simulink model "imu_model_with_submodules"  (R2015b)
settings: Solver=FixedStepAuto  StartTime=0.0  StopTime=10  FixedStep=1/mpu_sampling_frequency  RelTol=1e-3
values from neighbouring files (symbols this model uses):
  ex_acc_x = 0    [clipper.m]
  fs = mpu_sampling_frequency    [Madgwick_matlab.m]    (also in Mahony_matlab.m; clipper.m = 200)
  k = 0.05    [clipper.m]
  mpu_ax_noise_density = 300e-6    (= 0.0003)    [clipper.m]
  mpu_ax_sensitivity = 1/16384    (= 6.103515625e-05)    [clipper.m]
  mpu_ax_w = 460    [clipper.m]
  mpu_gyro_noise_density = 0.01    [clipper.m]
  mpu_gyro_sensitivity = 0.0610    (= 0.061)    [clipper.m]
  mpu_sampling_frequency = 200    [clipper.m]
  mpu_w = 250    [clipper.m]
undefined symbols (not defined in the file or in its folder): DiscIntNeverNeededParam, w_ax, wn, wn_ax, zeta, zeta_ax
libraries: simulink x9, aerolibtransform2 x2
settings Model: Creator=TOOsab  LastModifiedBy=TOOsab
settings DataIOCC: SaveOutput=off  SaveTime=off

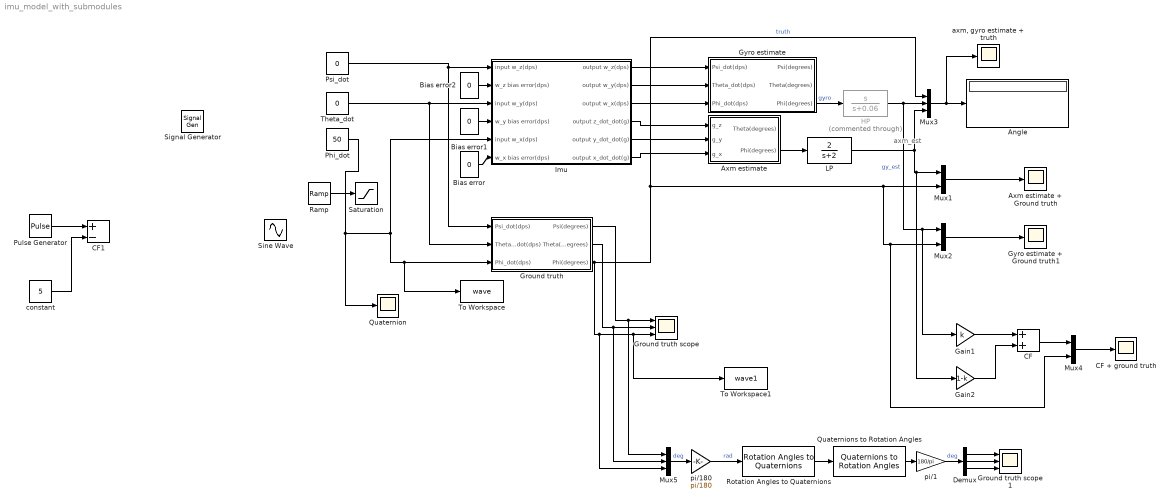
== system imu_model_with_submodules ==
  note: axm_est
  Angle : Display
  Axm estimate : Subsystem
  Axm estimate + Ground truth : Scope
  Bias error : Constant  Value=0
  Bias error1 : Constant  Value=0
  Bias error2 : Constant  Value=0
  CF : Sum
  CF + ground truth : Scope
  CF1 : Sum  Inputs=+-
  Demux : Demux  Outputs=3
  Gain1 : Gain  Gain=k
  Gain2 : Gain  Gain=1-k
  Ground truth : Subsystem
  "Ground truth scope " : Scope  NumInputPorts=3
  Ground truth scope 1 : Scope  NumInputPorts=3
  Gyro estimate : Subsystem
  Gyro estimate + Ground truth1 : Scope
  HP : TransferFcn  Commented=through  Numerator=[1 0]  Denominator=[1 0.06]
  Imu : Subsystem
  LP : TransferFcn  Numerator=[2]  Denominator=[1 2]
  Mux1 : Mux  Inputs=2
  Mux2 : Mux  Inputs=2
  Mux3 : Mux  Inputs=3
  Mux4 : Mux  Inputs=2
  Mux5 : Mux  Inputs=3
  Phi_dot : Constant  Value=50
  Psi_dot : Constant  Value=0
  Pulse Generator : DiscretePulseGenerator  PulseType=Time based  Amplitude=10  Period=10  PulseWidth=50
  Quaternion : Scope
  Quaternions to Rotation Angles : aerolibtransform2/Quaternions to Rotation Angles  rotationOrder=ZYX
  Ramp : simulink/Sources/Ramp  slope=1  start=1  X0=1
  Rotation Angles to Quaternions : aerolibtransform2/Rotation Angles to Quaternions  rotationOrder=ZYX
  Saturation : Saturate  UpperLimit=10
  Signal Generator : SignalGenerator  WaveForm=square  Frequency=0.1
  Sine Wave : Sin  Frequency=0.1  SampleTime=0
  Theta_dot : Constant  Value=0
  To Workspace : ToWorkspace  VariableName=wave  SampleTime=-1
  To Workspace1 : ToWorkspace  VariableName=wave1  SampleTime=-1
  "axm, gyro estimate + truth" : Scope
  constant : Constant  Value=5
  pi/1 : Gain  Gain=180/pi
  pi/180 : Gain  Gain=pi/180
  wires:
  Psi_dot/1 -> Ground truth/1(Psi_dot(dps)), Imu/1(input w_z(dps))
  Theta_dot/1 -> Ground truth/2(Theta_dot(dps)), Imu/3(input w_y(dps))
  Ramp/1 -> Saturation/1
  Imu/1(output w_z(dps)) -> Gyro estimate/1(Psi_dot(dps))
  Imu/2(output w_y(dps)) -> Gyro estimate/2(Theta_dot(dps))
  Imu/3(output w_x(dps)) -> Gyro estimate/3(Phi_dot(dps))
  Bias error/1 -> Imu/6(w_x bias error(dps))
  Ground truth/3(Phi(degrees)) -> Mux5/3, "Ground truth scope "/3, To Workspace1/1, Mux4/2, Mux2/2, Mux1/2, Mux3/1  "truth"
  Gyro estimate/3(Phi(degrees)) -> HP/1  "gyro"
  Mux3/1 -> Angle/1, "axm, gyro estimate + truth"/1
  Mux1/1 -> Axm estimate + Ground truth/1
  Bias error1/1 -> Imu/4(w_y bias error(dps))
  Bias error2/1 -> Imu/2(w_z bias error(dps))
  Imu/4(output z_dot_dot(g)) -> Axm estimate/1(g_z)
  Imu/5(output y_dot_dot(g)) -> Axm estimate/2(g_y)
  Imu/6(output x_dot_dot(g)) -> Axm estimate/3(g_x)
  Axm estimate/2(Phi(degrees)) -> LP/1
  LP/1 -> Gain2/1, Mux1/1, Mux3/3
  HP/1 -> Gain1/1, Mux2/1, Mux3/2  "gy_est"
  Mux2/1 -> Gyro estimate + Ground truth1/1
  Gain1/1 -> CF/1
  Gain2/1 -> CF/2
  CF/1 -> Mux4/1
  Mux4/1 -> CF + ground truth/1
  Ground truth/1(Psi(degrees)) -> "Ground truth scope "/1, Mux5/1
  Mux5/1 -> pi/180/1  "deg"
  Ground truth/2(Theta(degrees)) -> Mux5/2, "Ground truth scope "/2
  Rotation Angles to Quaternions/1 -> Quaternions to Rotation Angles/1
  Quaternions to Rotation Angles/1 -> pi/1/1
  Demux/1 -> Ground truth scope 1/1
  Demux/2 -> Ground truth scope 1/2
  Demux/3 -> Ground truth scope 1/3
  pi/180/1 -> Rotation Angles to Quaternions/1  "rad"
  pi/1/1 -> Demux/1  "deg"
  Phi_dot/1 -> Quaternion/1, Imu/5(input w_x(dps)), To Workspace/1, Ground truth/3(Phi_dot(dps))
  Pulse Generator/1 -> CF1/1
  constant/1 -> CF1/2

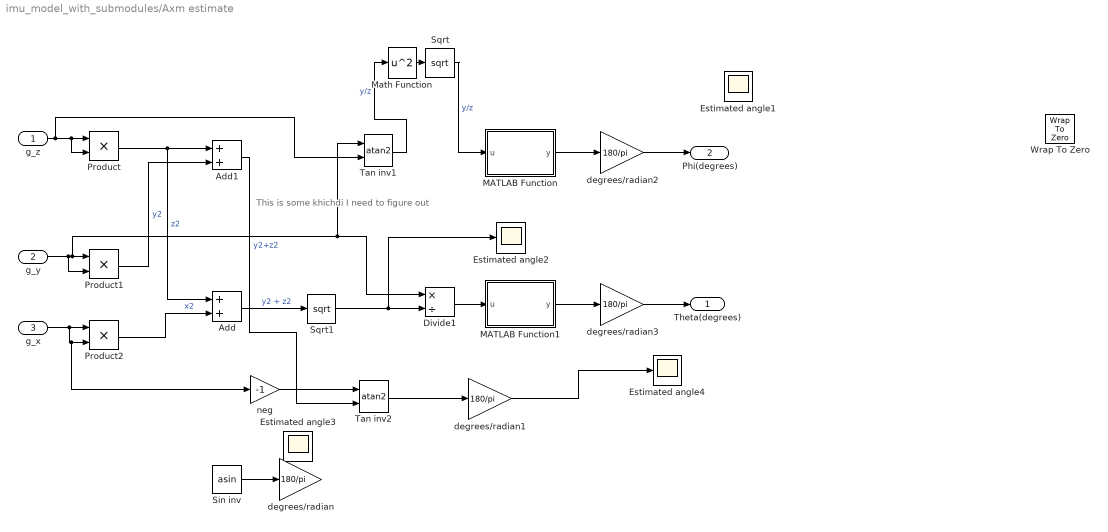
== system imu_model_with_submodules/Axm estimate ==
  note: This is some khichdi I need to figure out
  g_z : Inport
  g_y : Inport  Port=2
  g_x : Inport  Port=3
  Add : Sum
  Add1 : Sum
  Divide1 : Product  Inputs=*/
  Estimated angle{1..4} (4 alike) : Scope
  MATLAB Function : MATLAB Function  TreatAsAtomicUnit=on
  MATLAB Function1 : MATLAB Function  TreatAsAtomicUnit=on
  Math Function : Math  Operator=square  SaturateOnIntegerOverflow=on
  Product : Product
  Product1 : Product
  Product2 : Product
  Sin inv : Trigonometry  Operator=asin
  Sqrt : Sqrt  SaturateOnIntegerOverflow=on
  Sqrt1 : Sqrt  SaturateOnIntegerOverflow=on
  Tan inv1 : Trigonometry  Operator=atan2
  Tan inv2 : Trigonometry  Operator=atan2
  Wrap To Zero : simulink/Discontinuities/Wrap To Zero  Threshold=255
  degrees/radian{,1..3} (4 alike) : Gain  Gain=180/pi
  neg : Gain  Gain=-1
  Theta(degrees) : Outport
  Phi(degrees) : Outport  Port=2
  wires:
  Sin inv/1 -> degrees/radian/1
  g_z/1 -> Tan inv1/2, Product/2, Product/1
  g_y/1 -> Product1/2, Divide1/1, Tan inv1/1, Product1/1
  Product/1 -> Add/1, Add1/1  "z2"
  Product1/1 -> Add1/2  "y2"
  Product2/1 -> Add/2  "x2"
  Add/1 -> Sqrt1/1  "y2 + z2"
  Sqrt1/1 -> Estimated angle2/1, Divide1/2
  Divide1/1 -> MATLAB Function1/1(u)
  g_x/1 -> neg/1, Product2/2, Product2/1
  Add1/1 -> Tan inv2/2  "y2+z2"
  neg/1 -> Tan inv2/1
  Tan inv2/1 -> degrees/radian1/1
  degrees/radian1/1 -> Estimated angle4/1
  degrees/radian3/1 -> Theta(degrees)/1
  degrees/radian2/1 -> Phi(degrees)/1
  Sqrt/1 -> MATLAB Function/1(u)  "y/z"
  MATLAB Function/1(y) -> degrees/radian2/1
  MATLAB Function1/1(y) -> degrees/radian3/1
  Math Function/1 -> Sqrt/1
  Tan inv1/1 -> Math Function/1  "y/z"

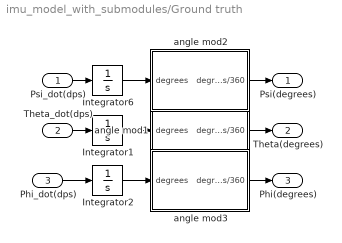
== system imu_model_with_submodules/Ground truth ==
  Psi_dot(dps) : Inport
  Theta_dot(dps) : Inport  Port=2
  Phi_dot(dps) : Inport  Port=3
  Integrator1 : Integrator
  Integrator2 : Integrator
  Integrator6 : Integrator
  angle mod1 : Subsystem
  angle mod2 : Subsystem
  angle mod3 : Subsystem
  Psi(degrees) : Outport
  Theta(degrees) : Outport  Port=2
  Phi(degrees) : Outport  Port=3
  wires:
  Phi_dot(dps)/1 -> Integrator2/1
  Integrator2/1 -> angle mod3/1(degrees)
  Theta_dot(dps)/1 -> Integrator1/1
  Psi_dot(dps)/1 -> Integrator6/1
  Integrator1/1 -> angle mod1/1(degrees)
  Integrator6/1 -> angle mod2/1(degrees)
  angle mod2/1(degrees/360) -> Psi(degrees)/1
  angle mod1/1(degrees/360) -> Theta(degrees)/1
  angle mod3/1(degrees/360) -> Phi(degrees)/1

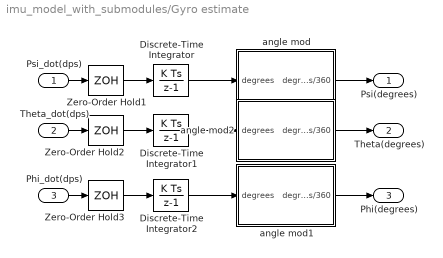
== system imu_model_with_submodules/Gyro estimate ==
  Psi_dot(dps) : Inport
  Theta_dot(dps) : Inport  Port=2
  Phi_dot(dps) : Inport  Port=3
  Discrete-Time Integrator : DiscreteIntegrator  InitialConditionSetting=State (most efficient)  SampleTime=1/mpu_sampling_frequency  ICPrevOutput=DiscIntNeverNeededParam  ICPrevScaledInput=DiscIntNeverNeededParam
  Discrete-Time Integrator1 : DiscreteIntegrator  InitialConditionSetting=State (most efficient)  SampleTime=1/mpu_sampling_frequency  ICPrevOutput=DiscIntNeverNeededParam  ICPrevScaledInput=DiscIntNeverNeededParam
  Discrete-Time Integrator2 : DiscreteIntegrator  InitialConditionSetting=State (most efficient)  SampleTime=1/mpu_sampling_frequency  ICPrevOutput=DiscIntNeverNeededParam  ICPrevScaledInput=DiscIntNeverNeededParam
  Zero-Order Hold1 : ZeroOrderHold  SampleTime=1/mpu_sampling_frequency
  Zero-Order Hold2 : ZeroOrderHold  SampleTime=1/mpu_sampling_frequency
  Zero-Order Hold3 : ZeroOrderHold  SampleTime=1/mpu_sampling_frequency
  angle mod : Subsystem
  angle mod1 : Subsystem
  angle mod2 : Subsystem
  Psi(degrees) : Outport
  Theta(degrees) : Outport  Port=2
  Phi(degrees) : Outport  Port=3
  wires:
  Zero-Order Hold1/1 -> Discrete-Time Integrator/1
  Zero-Order Hold3/1 -> Discrete-Time Integrator2/1
  Zero-Order Hold2/1 -> Discrete-Time Integrator1/1
  Discrete-Time Integrator2/1 -> angle mod1/1(degrees)
  Phi_dot(dps)/1 -> Zero-Order Hold3/1
  Discrete-Time Integrator/1 -> angle mod/1(degrees)
  Discrete-Time Integrator1/1 -> angle mod2/1(degrees)
  Psi_dot(dps)/1 -> Zero-Order Hold1/1
  Theta_dot(dps)/1 -> Zero-Order Hold2/1
  angle mod/1(degrees/360) -> Psi(degrees)/1
  angle mod2/1(degrees/360) -> Theta(degrees)/1
  angle mod1/1(degrees/360) -> Phi(degrees)/1

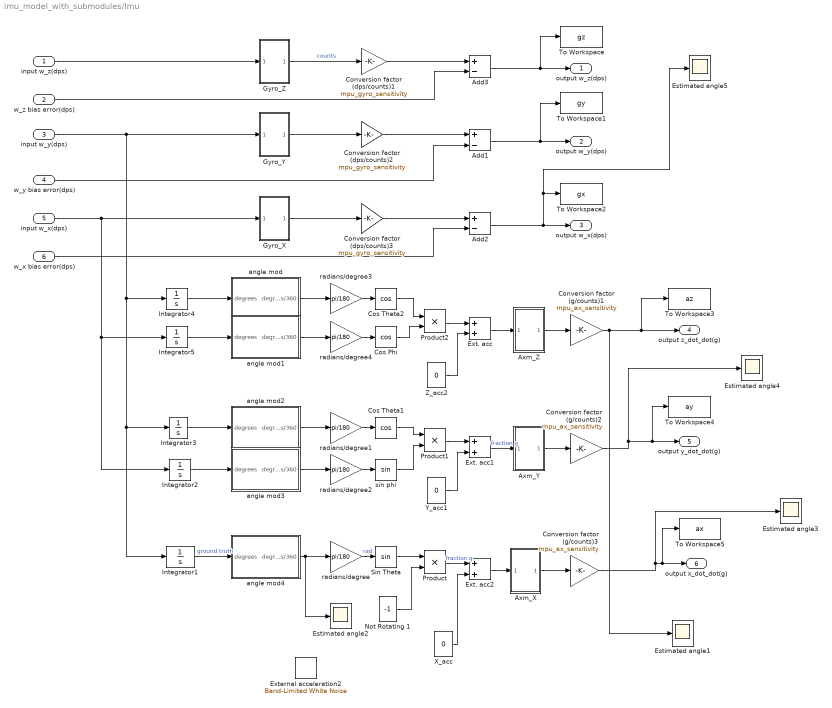
== system imu_model_with_submodules/Imu ==
  input w_z(dps) : Inport
  w_z bias error(dps) : Inport  Port=2
  input w_y(dps) : Inport  Port=3
  w_y bias error(dps) : Inport  Port=4
  input w_x(dps) : Inport  Port=5
  w_x bias error(dps) : Inport  Port=6
  Add1 : Sum  Inputs=+-
  Add2 : Sum  Inputs=+-
  Add3 : Sum  Inputs=+-
  Axm_X : Subsystem
  Axm_Y : Subsystem
  Axm_Z : Subsystem
  Conversion factor (dps/counts)1 : Gain  Gain=mpu_gyro_sensitivity
  Conversion factor (dps/counts)2 : Gain  Gain=mpu_gyro_sensitivity
  Conversion factor (dps/counts)3 : Gain  Gain=mpu_gyro_sensitivity
  Conversion factor (g/counts)1 : Gain  Gain=mpu_ax_sensitivity
  Conversion factor (g/counts)2 : Gain  Gain=mpu_ax_sensitivity
  Conversion factor (g/counts)3 : Gain  Gain=mpu_ax_sensitivity
  Cos Phi : Trigonometry  Operator=cos
  Cos Theta1 : Trigonometry  Operator=cos
  Cos Theta2 : Trigonometry  Operator=cos
  Estimated angle{1..5} (5 alike) : Scope
  Ext. acc : Sum
  Ext. acc1 : Sum
  Ext. acc2 : Sum
  External acceleration2 : simulink/Sources/Band-Limited White Noise  Cov=[ex_acc_x]  Ts=1/fs  seed=[23341]
  Gyro_X : Subsystem
  Gyro_Y : Subsystem
  Gyro_Z : Subsystem
  Integrator{1..5} (5 alike) : Integrator
  Not Rotating 1 : Constant  Value=-1
  Product : Product
  Product1 : Product
  Product2 : Product
  Sin Theta : Trigonometry
  To Workspace : ToWorkspace  VariableName=gz  SampleTime=-1
  To Workspace1 : ToWorkspace  VariableName=gy  SampleTime=-1
  To Workspace2 : ToWorkspace  VariableName=gx  SampleTime=-1
  To Workspace3 : ToWorkspace  VariableName=az  SampleTime=-1
  To Workspace4 : ToWorkspace  VariableName=ay  SampleTime=-1
  To Workspace5 : ToWorkspace  VariableName=ax  SampleTime=-1
  X_acc : Constant  Value=0
  Y_acc1 : Constant  Value=0
  Z_acc2 : Constant  Value=0
  angle mod : Subsystem
  angle mod1 : Subsystem
  angle mod2 : Subsystem
  angle mod3 : Subsystem
  angle mod4 : Subsystem
  radians/degree{,1..4} (5 alike) : Gain  Gain=pi/180
  sin phi : Trigonometry
  output w_z(dps) : Outport
  output w_y(dps) : Outport  Port=2
  output w_x(dps) : Outport  Port=3
  output z_dot_dot(g) : Outport  Port=4
  output y_dot_dot(g) : Outport  Port=5
  output x_dot_dot(g) : Outport  Port=6
  wires:
  input w_y(dps)/1 -> Integrator4/1, Integrator3/1, Integrator1/1, Gyro_Y/1(In1)
  Gyro_X/1(Out1) -> Conversion factor (dps/counts)3/1
  Gyro_Y/1(Out1) -> Conversion factor (dps/counts)2/1
  Gyro_Z/1(Out1) -> Conversion factor (dps/counts)1/1  "counts"
  input w_x(dps)/1 -> Integrator2/1, Integrator5/1, Gyro_X/1(In1)
  Conversion factor (dps/counts)2/1 -> Add1/1
  Add2/1 -> Estimated angle5/1, To Workspace2/1, output w_x(dps)/1
  Add3/1 -> To Workspace/1, output w_z(dps)/1
  Conversion factor (dps/counts)3/1 -> Add2/1
  Add1/1 -> To Workspace1/1, output w_y(dps)/1
  Conversion factor (dps/counts)1/1 -> Add3/1
  w_z bias error(dps)/1 -> Add3/2
  w_y bias error(dps)/1 -> Add1/2
  w_x bias error(dps)/1 -> Add2/2
  Integrator4/1 -> angle mod/1(degrees)
  radians/degree3/1 -> Cos Theta2/1
  Cos Theta2/1 -> Product2/1
  Integrator5/1 -> angle mod1/1(degrees)
  radians/degree4/1 -> Cos Phi/1
  Cos Phi/1 -> Product2/2
  Axm_Z/1(Out1) -> Conversion factor (g/counts)1/1
  Product2/1 -> Ext. acc/1
  Ext. acc1/1 -> Axm_Y/1(In1)  "fraction g"
  Axm_Y/1(Out1) -> Conversion factor (g/counts)2/1
  Integrator3/1 -> angle mod2/1(degrees)
  Integrator2/1 -> angle mod3/1(degrees)
  radians/degree1/1 -> Cos Theta1/1
  radians/degree2/1 -> sin phi/1
  Cos Theta1/1 -> Product1/1
  sin phi/1 -> Product1/2
  Sin Theta/1 -> Product/1
  Not Rotating 1/1 -> Product/2
  radians/degree/1 -> Sin Theta/1  "rad"
  Integrator1/1 -> angle mod4/1(degrees)  "ground truth"
  Axm_X/1(Out1) -> Conversion factor (g/counts)3/1
  Product/1 -> Ext. acc2/1  "fraction g"
  input w_z(dps)/1 -> Gyro_Z/1(In1)
  Conversion factor (g/counts)3/1 -> Estimated angle3/1, To Workspace5/1, output x_dot_dot(g)/1
  Conversion factor (g/counts)1/1 -> Estimated angle1/1, To Workspace3/1, output z_dot_dot(g)/1
  angle mod/1(degrees/360) -> radians/degree3/1
  angle mod1/1(degrees/360) -> radians/degree4/1
  angle mod2/1(degrees/360) -> radians/degree1/1
  angle mod3/1(degrees/360) -> radians/degree2/1
  angle mod4/1(degrees/360) -> Estimated angle2/1, radians/degree/1
  Conversion factor (g/counts)2/1 -> Estimated angle4/1, To Workspace4/1, output y_dot_dot(g)/1
  Ext. acc/1 -> Axm_Z/1(In1)
  Product1/1 -> Ext. acc1/1
  X_acc/1 -> Ext. acc2/2
  Ext. acc2/1 -> Axm_X/1(In1)
  Y_acc1/1 -> Ext. acc1/2
  Z_acc2/1 -> Ext. acc/2

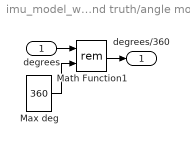
== system imu_model_with_submodules/Ground truth/angle mod1 ==
  degrees : Inport
  Math Function1 : Math  Operator=rem  RndMeth=Zero  SaturateOnIntegerOverflow=on
  Max deg : Constant  Value=360
  degrees/360 : Outport
  wires:
  degrees/1 -> Math Function1/1
  Max deg/1 -> Math Function1/2
  Math Function1/1 -> degrees/360/1

== system imu_model_with_submodules/Ground truth/angle mod2 ==
  degrees : Inport
  Math Function1 : Math  Operator=rem  RndMeth=Zero  SaturateOnIntegerOverflow=on
  Max deg : Constant  Value=360
  degrees/360 : Outport
  wires:
  degrees/1 -> Math Function1/1
  Max deg/1 -> Math Function1/2
  Math Function1/1 -> degrees/360/1

== system imu_model_with_submodules/Ground truth/angle mod3 ==
  degrees : Inport
  Math Function1 : Math  Operator=rem  RndMeth=Zero  SaturateOnIntegerOverflow=on
  Max deg : Constant  Value=360
  degrees/360 : Outport
  wires:
  degrees/1 -> Math Function1/1
  Max deg/1 -> Math Function1/2
  Math Function1/1 -> degrees/360/1

== system imu_model_with_submodules/Gyro estimate/angle mod ==
  degrees : Inport
  Math Function1 : Math  Operator=rem  RndMeth=Zero  SaturateOnIntegerOverflow=on
  Max deg : Constant  Value=360
  degrees/360 : Outport
  wires:
  degrees/1 -> Math Function1/1
  Max deg/1 -> Math Function1/2
  Math Function1/1 -> degrees/360/1

== system imu_model_with_submodules/Gyro estimate/angle mod1 ==
  degrees : Inport
  Math Function1 : Math  Operator=rem  RndMeth=Zero  SaturateOnIntegerOverflow=on
  Max deg : Constant  Value=360
  degrees/360 : Outport
  wires:
  degrees/1 -> Math Function1/1
  Max deg/1 -> Math Function1/2
  Math Function1/1 -> degrees/360/1

== system imu_model_with_submodules/Gyro estimate/angle mod2 ==
  degrees : Inport
  Math Function1 : Math  Operator=rem  RndMeth=Zero  SaturateOnIntegerOverflow=on
  Max deg : Constant  Value=360
  degrees/360 : Outport
  wires:
  degrees/1 -> Math Function1/1
  Max deg/1 -> Math Function1/2
  Math Function1/1 -> degrees/360/1

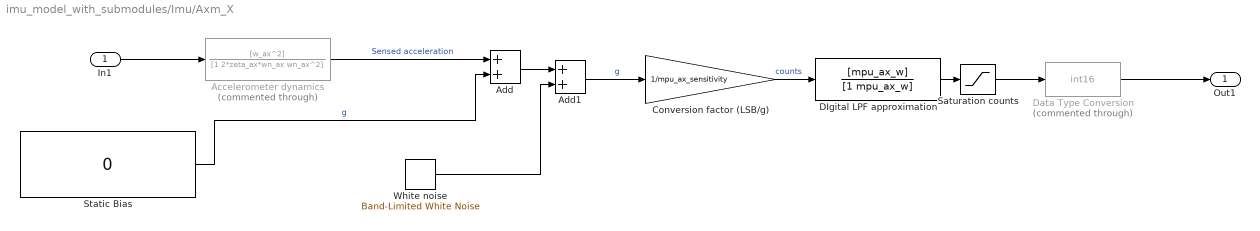
== system imu_model_with_submodules/Imu/Axm_X ==
  In1 : Inport
  Accelerometer dynamics : TransferFcn  Commented=through  Numerator=[w_ax^2]  Denominator=[1 2*zeta_ax*wn_ax wn_ax^2]
  Add : Sum
  Add1 : Sum
  Conversion factor (LSB/g) : Gain  Gain=1/mpu_ax_sensitivity
  DIgital LPF approximation : TransferFcn  Numerator=[mpu_ax_w]  Denominator=[1 mpu_ax_w]
  Data Type Conversion : DataTypeConversion  Commented=through  OutDataTypeStr=int16
  "Saturation counts " : Saturate  UpperLimit=2^15  LowerLimit=-2^15
  Static Bias : Constant  Value=0
  White noise : simulink/Sources/Band-Limited White Noise  Cov=[(mpu_ax_noise_density)^2]  Ts=1/mpu_sampling_frequency  seed=[23341]
  Out1 : Outport
  wires:
  In1/1 -> Accelerometer dynamics/1
  Data Type Conversion/1 -> Out1/1
  "Saturation counts "/1 -> Data Type Conversion/1
  DIgital LPF approximation/1 -> "Saturation counts "/1
  Add1/1 -> Conversion factor (LSB/g)/1  "g"
  Add/1 -> Add1/1
  White noise/1 -> Add1/2
  Accelerometer dynamics/1 -> Add/1  "Sensed acceleration"
  Static Bias/1 -> Add/2  "g"
  Conversion factor (LSB/g)/1 -> DIgital LPF approximation/1  "counts"

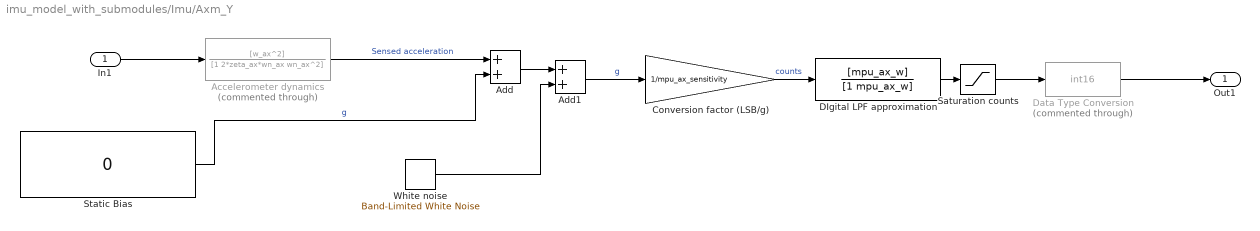
== system imu_model_with_submodules/Imu/Axm_Y ==
  In1 : Inport
  Accelerometer dynamics : TransferFcn  Commented=through  Numerator=[w_ax^2]  Denominator=[1 2*zeta_ax*wn_ax wn_ax^2]
  Add : Sum
  Add1 : Sum
  Conversion factor (LSB/g) : Gain  Gain=1/mpu_ax_sensitivity
  DIgital LPF approximation : TransferFcn  Numerator=[mpu_ax_w]  Denominator=[1 mpu_ax_w]
  Data Type Conversion : DataTypeConversion  Commented=through  OutDataTypeStr=int16
  "Saturation counts " : Saturate  UpperLimit=2^15  LowerLimit=-2^15
  Static Bias : Constant  Value=0
  White noise : simulink/Sources/Band-Limited White Noise  Cov=[(mpu_ax_noise_density)^2]  Ts=1/mpu_sampling_frequency  seed=[23341]
  Out1 : Outport
  wires:
  In1/1 -> Accelerometer dynamics/1
  Data Type Conversion/1 -> Out1/1
  "Saturation counts "/1 -> Data Type Conversion/1
  DIgital LPF approximation/1 -> "Saturation counts "/1
  Add1/1 -> Conversion factor (LSB/g)/1  "g"
  Add/1 -> Add1/1
  White noise/1 -> Add1/2
  Accelerometer dynamics/1 -> Add/1  "Sensed acceleration"
  Static Bias/1 -> Add/2  "g"
  Conversion factor (LSB/g)/1 -> DIgital LPF approximation/1  "counts"

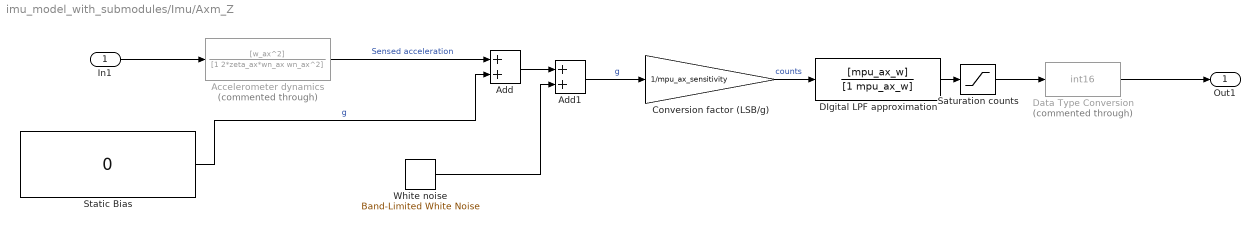
== system imu_model_with_submodules/Imu/Axm_Z ==
  In1 : Inport
  Accelerometer dynamics : TransferFcn  Commented=through  Numerator=[w_ax^2]  Denominator=[1 2*zeta_ax*wn_ax wn_ax^2]
  Add : Sum
  Add1 : Sum
  Conversion factor (LSB/g) : Gain  Gain=1/mpu_ax_sensitivity
  DIgital LPF approximation : TransferFcn  Numerator=[mpu_ax_w]  Denominator=[1 mpu_ax_w]
  Data Type Conversion : DataTypeConversion  Commented=through  OutDataTypeStr=int16
  "Saturation counts " : Saturate  UpperLimit=2^15  LowerLimit=-2^15
  Static Bias : Constant  Value=0
  White noise : simulink/Sources/Band-Limited White Noise  Cov=[(mpu_ax_noise_density)^2]  Ts=1/mpu_sampling_frequency  seed=[23341]
  Out1 : Outport
  wires:
  In1/1 -> Accelerometer dynamics/1
  Data Type Conversion/1 -> Out1/1
  "Saturation counts "/1 -> Data Type Conversion/1
  DIgital LPF approximation/1 -> "Saturation counts "/1
  Add1/1 -> Conversion factor (LSB/g)/1  "g"
  Add/1 -> Add1/1
  White noise/1 -> Add1/2
  Accelerometer dynamics/1 -> Add/1  "Sensed acceleration"
  Static Bias/1 -> Add/2  "g"
  Conversion factor (LSB/g)/1 -> DIgital LPF approximation/1  "counts"

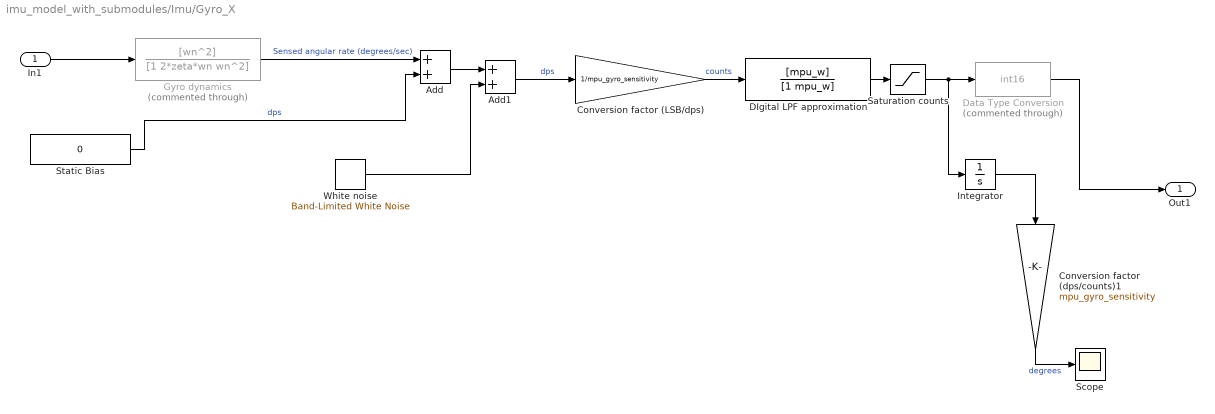
== system imu_model_with_submodules/Imu/Gyro_X ==
  In1 : Inport
  Add : Sum
  Add1 : Sum
  Conversion factor (LSB/dps) : Gain  Gain=1/mpu_gyro_sensitivity
  Conversion factor (dps/counts)1 : Gain  Gain=mpu_gyro_sensitivity
  DIgital LPF approximation : TransferFcn  Numerator=[mpu_w]  Denominator=[1 mpu_w]
  Data Type Conversion : DataTypeConversion  Commented=through  OutDataTypeStr=int16
  Gyro dynamics : TransferFcn  Commented=through  Numerator=[wn^2]  Denominator=[1 2*zeta*wn wn^2]
  Integrator : Integrator
  "Saturation counts " : Saturate  UpperLimit=2^15  LowerLimit=-2^15
  Scope : Scope
  Static Bias : Constant  Value=0
  White noise : simulink/Sources/Band-Limited White Noise  Cov=[(mpu_gyro_noise_density)^2]  Ts=1/mpu_sampling_frequency  seed=[23341]
  Out1 : Outport
  wires:
  Gyro dynamics/1 -> Add/1  "Sensed angular rate (degrees/sec)"
  White noise/1 -> Add1/2
  Static Bias/1 -> Add/2  "dps"
  Conversion factor (LSB/dps)/1 -> DIgital LPF approximation/1  "counts"
  Add/1 -> Add1/1
  Conversion factor (dps/counts)1/1 -> Scope/1  "degrees"
  Integrator/1 -> Conversion factor (dps/counts)1/1
  Data Type Conversion/1 -> Out1/1
  In1/1 -> Gyro dynamics/1
  "Saturation counts "/1 -> Integrator/1, Data Type Conversion/1
  DIgital LPF approximation/1 -> "Saturation counts "/1
  Add1/1 -> Conversion factor (LSB/dps)/1  "dps"

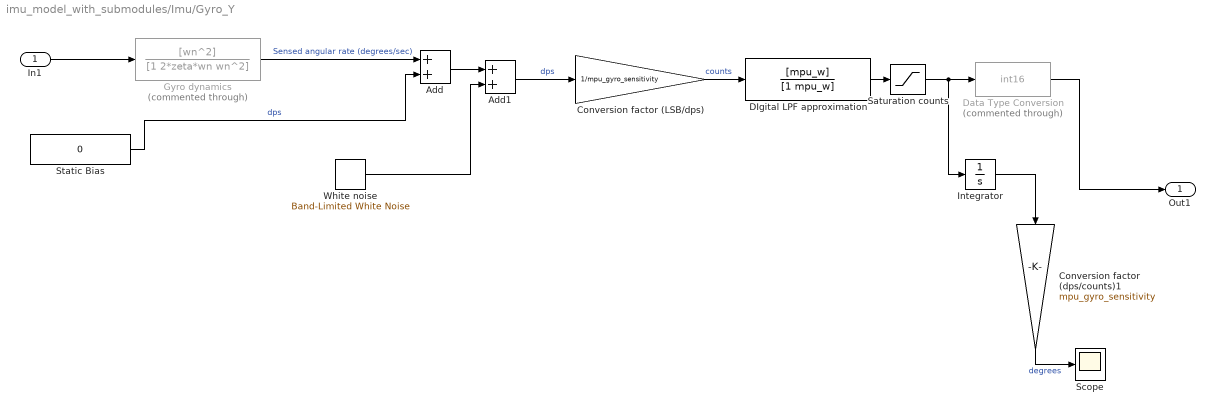
== system imu_model_with_submodules/Imu/Gyro_Y ==
  In1 : Inport
  Add : Sum
  Add1 : Sum
  Conversion factor (LSB/dps) : Gain  Gain=1/mpu_gyro_sensitivity
  Conversion factor (dps/counts)1 : Gain  Gain=mpu_gyro_sensitivity
  DIgital LPF approximation : TransferFcn  Numerator=[mpu_w]  Denominator=[1 mpu_w]
  Data Type Conversion : DataTypeConversion  Commented=through  OutDataTypeStr=int16
  Gyro dynamics : TransferFcn  Commented=through  Numerator=[wn^2]  Denominator=[1 2*zeta*wn wn^2]
  Integrator : Integrator
  "Saturation counts " : Saturate  UpperLimit=2^15  LowerLimit=-2^15
  Scope : Scope
  Static Bias : Constant  Value=0
  White noise : simulink/Sources/Band-Limited White Noise  Cov=[(mpu_gyro_noise_density)^2]  Ts=1/mpu_sampling_frequency  seed=[23341]
  Out1 : Outport
  wires:
  Add1/1 -> Conversion factor (LSB/dps)/1  "dps"
  DIgital LPF approximation/1 -> "Saturation counts "/1
  "Saturation counts "/1 -> Data Type Conversion/1, Integrator/1
  In1/1 -> Gyro dynamics/1
  Data Type Conversion/1 -> Out1/1
  Integrator/1 -> Conversion factor (dps/counts)1/1
  Conversion factor (dps/counts)1/1 -> Scope/1  "degrees"
  Add/1 -> Add1/1
  Conversion factor (LSB/dps)/1 -> DIgital LPF approximation/1  "counts"
  Static Bias/1 -> Add/2  "dps"
  White noise/1 -> Add1/2
  Gyro dynamics/1 -> Add/1  "Sensed angular rate (degrees/sec)"

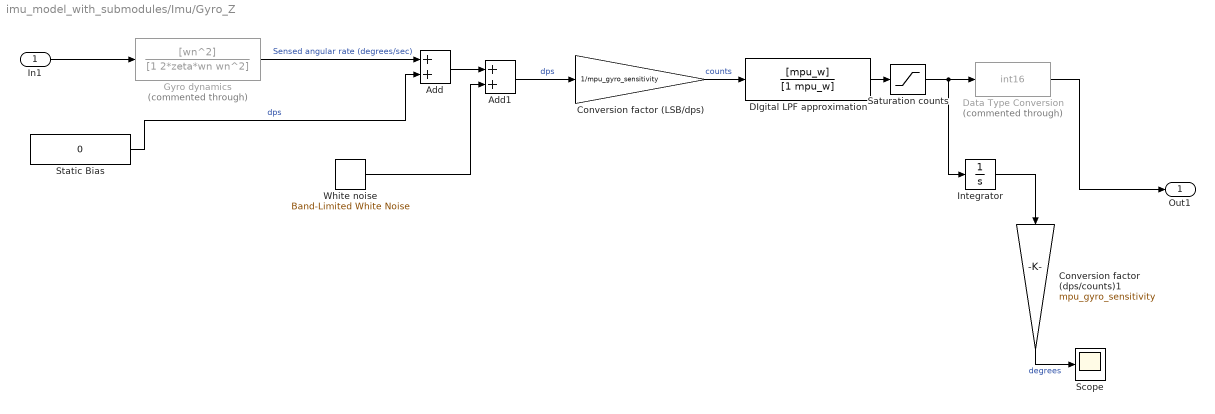
== system imu_model_with_submodules/Imu/Gyro_Z ==
  In1 : Inport
  Add : Sum
  Add1 : Sum
  Conversion factor (LSB/dps) : Gain  Gain=1/mpu_gyro_sensitivity
  Conversion factor (dps/counts)1 : Gain  Gain=mpu_gyro_sensitivity
  DIgital LPF approximation : TransferFcn  Numerator=[mpu_w]  Denominator=[1 mpu_w]
  Data Type Conversion : DataTypeConversion  Commented=through  OutDataTypeStr=int16
  Gyro dynamics : TransferFcn  Commented=through  Numerator=[wn^2]  Denominator=[1 2*zeta*wn wn^2]
  Integrator : Integrator
  "Saturation counts " : Saturate  UpperLimit=2^15  LowerLimit=-2^15
  Scope : Scope
  Static Bias : Constant  Value=0
  White noise : simulink/Sources/Band-Limited White Noise  Cov=[(mpu_gyro_noise_density)^2]  Ts=1/mpu_sampling_frequency  seed=[23341]
  Out1 : Outport
  wires:
  Gyro dynamics/1 -> Add/1  "Sensed angular rate (degrees/sec)"
  White noise/1 -> Add1/2
  Static Bias/1 -> Add/2  "dps"
  Conversion factor (LSB/dps)/1 -> DIgital LPF approximation/1  "counts"
  Add/1 -> Add1/1
  Conversion factor (dps/counts)1/1 -> Scope/1  "degrees"
  Integrator/1 -> Conversion factor (dps/counts)1/1
  Data Type Conversion/1 -> Out1/1
  In1/1 -> Gyro dynamics/1
  "Saturation counts "/1 -> Integrator/1, Data Type Conversion/1
  DIgital LPF approximation/1 -> "Saturation counts "/1
  Add1/1 -> Conversion factor (LSB/dps)/1  "dps"

== system imu_model_with_submodules/Imu/angle mod ==
  degrees : Inport
  Math Function1 : Math  Operator=rem  RndMeth=Zero  SaturateOnIntegerOverflow=on
  Max deg : Constant  Value=360
  degrees/360 : Outport
  wires:
  degrees/1 -> Math Function1/1
  Max deg/1 -> Math Function1/2
  Math Function1/1 -> degrees/360/1

== system imu_model_with_submodules/Imu/angle mod1 ==
  degrees : Inport
  Math Function1 : Math  Operator=rem  RndMeth=Zero  SaturateOnIntegerOverflow=on
  Max deg : Constant  Value=360
  degrees/360 : Outport
  wires:
  Math Function1/1 -> degrees/360/1
  Max deg/1 -> Math Function1/2
  degrees/1 -> Math Function1/1

== system imu_model_with_submodules/Imu/angle mod2 ==
  degrees : Inport
  Math Function1 : Math  Operator=rem  RndMeth=Zero  SaturateOnIntegerOverflow=on
  Max deg : Constant  Value=360
  degrees/360 : Outport
  wires:
  degrees/1 -> Math Function1/1
  Max deg/1 -> Math Function1/2
  Math Function1/1 -> degrees/360/1

== system imu_model_with_submodules/Imu/angle mod3 ==
  degrees : Inport
  Math Function1 : Math  Operator=rem  RndMeth=Zero  SaturateOnIntegerOverflow=on
  Max deg : Constant  Value=360
  degrees/360 : Outport
  wires:
  Math Function1/1 -> degrees/360/1
  Max deg/1 -> Math Function1/2
  degrees/1 -> Math Function1/1

== system imu_model_with_submodules/Imu/angle mod4 ==
  degrees : Inport
  Math Function1 : Math  Operator=rem  RndMeth=Zero  SaturateOnIntegerOverflow=on
  Max deg : Constant  Value=360
  degrees/360 : Outport
  wires:
  degrees/1 -> Math Function1/1
  Max deg/1 -> Math Function1/2
  Math Function1/1 -> degrees/360/1

== matlab function imu_model_with_submodules/Axm estimate/MATLAB Function ==
  data: u input; y output
function y = fcn(u)
%#codegen
y = coder.nullcopy(zeros(size(u)));
coder.extrinsic('wrapTo2Pi');
y = wrapTo2Pi(u);

== matlab function imu_model_with_submodules/Axm estimate/MATLAB Function1 ==
  data: u input; y output
function y = fcn(u)
%#codegen
y = coder.nullcopy(zeros(size(u)));
coder.extrinsic('wrapTo2Pi');
y = wrapTo2Pi(u);
